simulink model "Simulation"  (R2023b)
settings: Solver=VariableStepAuto  StartTime=0.0  StopTime=10.0  RelTol=1e-3
InitFcn:
  | init_param
values from neighbouring files (symbols this model uses):
  dtheta_0 = 0    [init_param.m]
  dxc_0 = 0    [init_param.m]
  r = 0.1    [init_param.m]
  theta_0 = pi/3    (= 1.0471975512)    [init_param.m]
  xc_0 = 2    [init_param.m]
undefined symbols (not defined in the file or in its folder): dim, std_dev, Ts
settings Model: Creator=rvitt  LastModifiedBy=franc
settings OptimizationCC: ReuseModelBlockBuffer=off

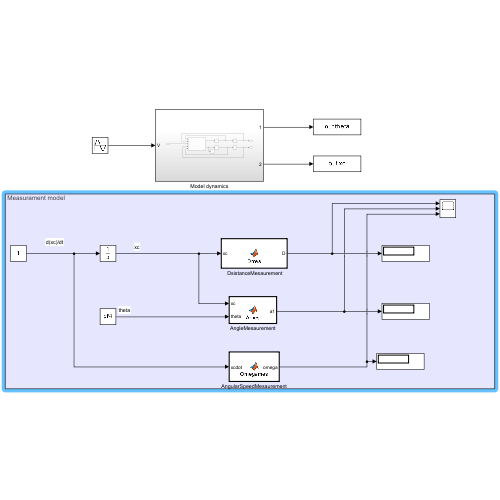
[thumbnail: Simulink's stored preview of the top-level diagram]
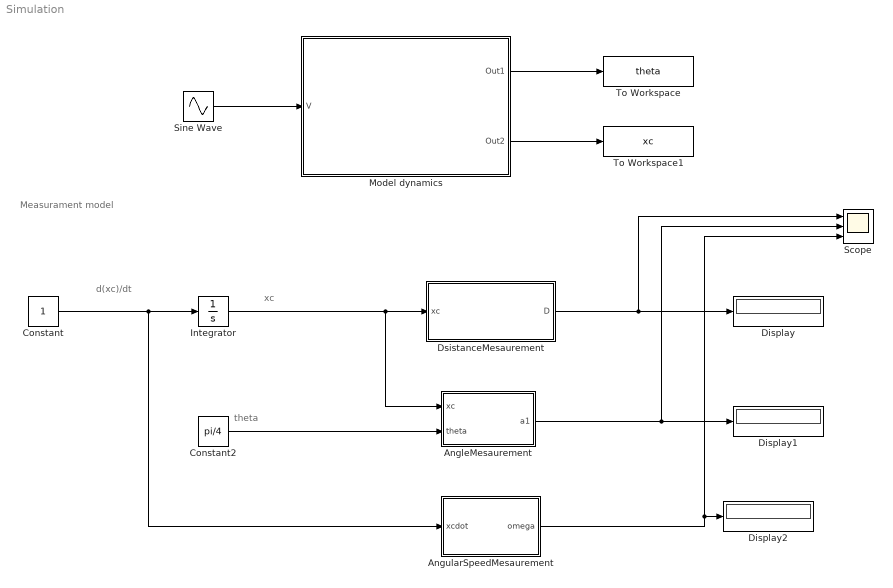
== system Simulation ==
  note: Measurament model
  note: d(xc)/dt
  note: xc
  note: theta
  " DsistanceMesaurement" : MATLAB Function  TreatAsAtomicUnit=on  SystemSampleTime=Ts.distance_sensor
  AngleMesaurement : MATLAB Function  TreatAsAtomicUnit=on  SystemSampleTime=Ts.a1_sensor
  AngularSpeedMesaurement : MATLAB Function  TreatAsAtomicUnit=on  SystemSampleTime=Ts.angularspeed_sensor
  Constant : Constant
  Constant2 : Constant  Value=pi/4
  Display : Display
  Display1 : Display
  Display2 : Display
  Integrator : Integrator
  Model dynamics : Subsystem
  Scope : Scope  NumInputPorts=3
  Sine Wave : Sin  Amplitude=50  SampleTime=0
  To Workspace : ToWorkspace  VariableName=theta  SaveFormat=Timeseries  SampleTime=-1
  To Workspace1 : ToWorkspace  VariableName=xc  SaveFormat=Timeseries  SampleTime=-1
  wires:
  Model dynamics/1(Out1) -> To Workspace/1
  Model dynamics/2(Out2) -> To Workspace1/1
  Sine Wave/1 -> Model dynamics/1(V)
  Constant2/1 -> AngleMesaurement/2(theta)
  AngularSpeedMesaurement/1(omega) -> Scope/3, Display2/1
  AngleMesaurement/1(a1) -> Display1/1, Scope/2
  Constant/1 -> AngularSpeedMesaurement/1(xcdot), Integrator/1
  Integrator/1 -> " DsistanceMesaurement"/1(xc), AngleMesaurement/1(xc)
  " DsistanceMesaurement"/1(D) -> Scope/1, Display/1

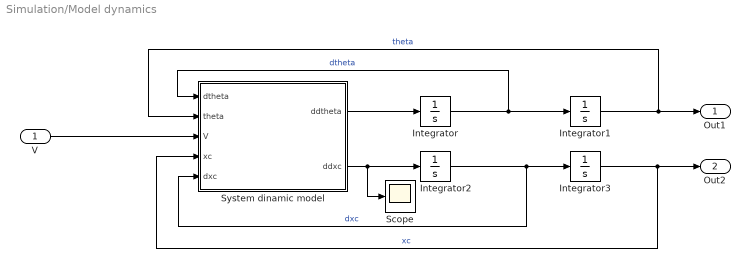
== system Simulation/Model dynamics ==
  V : Inport
  Integrator : Integrator  InitialCondition=dtheta_0
  Integrator1 : Integrator  InitialCondition=theta_0
  Integrator2 : Integrator  InitialCondition=dxc_0
  Integrator3 : Integrator  InitialCondition=xc_0
  Scope : Scope
  System dinamic model : MATLAB Function  TreatAsAtomicUnit=on
  Out1 : Outport
  Out2 : Outport  Port=2
  wires:
  Integrator/1 -> System dinamic model/1(dtheta), Integrator1/1  "dtheta"
  Integrator2/1 -> System dinamic model/5(dxc), Integrator3/1  "dxc"
  System dinamic model/1(ddtheta) -> Integrator/1
  System dinamic model/2(ddxc) -> Scope/1, Integrator2/1
  Integrator3/1 -> System dinamic model/4(xc), Out2/1  "xc"
  Integrator1/1 -> Out1/1, System dinamic model/2(theta)  "theta"
  V/1 -> System dinamic model/3(V)

== matlab function Simulation/ DsistanceMesaurement ==
  data: D output; xc input; dim parameter; std_dev parameter
function D = Dmes(xc, dim, std_dev)

D = (dim.xmax - dim.xmin) - xc + std_dev.distance_sensor*randn(1,1);

end

== matlab function Simulation/Model dynamics/System dinamic model ==
  data: dtheta input; theta input; V input; ddtheta output; xc input; dxc input; param parameter; ddxc output
function [ddtheta, ddxc] = fcn(dtheta, theta, V, xc, dxc, param)

% Rename variable
M = param.M;
N = param.N;
P = param.P;
W = param.W;
Rm = param.Rm;

g = 9.81;       % [m/s^2] 


% Dynam equations
ddxc = (V*N*M - dxc*N*W^2 + cos(theta)*g*sin(theta)*Rm*P^2 + dtheta^2*sin(theta)*Rm*N*P)/(Rm*(N*M - cos(theta)^2*P^2));

ddtheta = - P/Rm * (g*sin(theta)*Rm*M + cos(theta)*dtheta^2*sin(theta)*Rm*P + cos(theta)*V*M - cos(theta)*dxc*W^2)/(N*M - cos(theta)^2*P^2);

== matlab function Simulation/AngleMesaurement ==
  data: a1 output; xc input; theta input; dim parameter; std_dev parameter
function a1 = Ames(xc, theta, dim, std_dev)

a1 = atan2(-dim.Lp*cos(theta), xc + dim.Lp*sin(theta)) + std_dev.a1_sensor*randn(1,1);

end

== matlab function Simulation/AngularSpeedMesaurement ==
  data: xcdot input; omega output; r parameter; std_dev parameter
function omega = Omegames(xcdot, r, std_dev)

omega = 2*xcdot/r + std_dev.angularspeed_sensor*randn(1, 1);

end
